simulink model "Top_Level"  (Simulink 7.5)
settings: Solver=ode45  StartTime=0.0  StopTime=inf  RelTol=1e-3
undefined symbols (not defined in the file): dfilt, DiscIntNeverNeededParam, fspecial, gray, Horn, imresize, Low, Rec, Schunck, SDTV
libraries: simulink x13, dspobslib x10, dspsigops x4, vipgeotforms x4, viptextngfix x4, vipsnks x3, dspmtrx3 x2, vipanalysis x2, vipconversions x1, dsparch4 x1, dspswit3 x1, vipsrcs x1
(part 2 of 2)

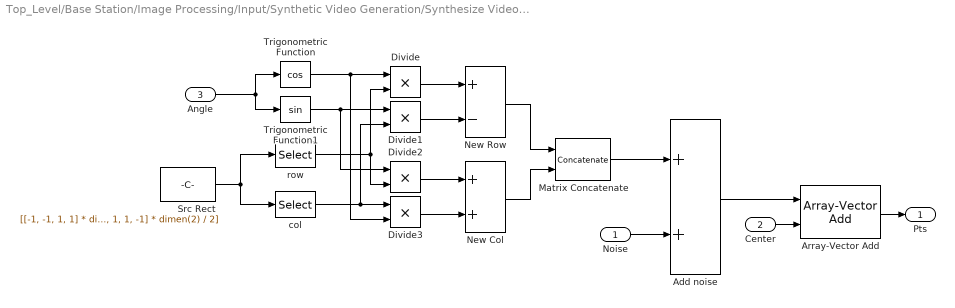
== system Top_Level/Base Station/Image Processing/Input/Synthetic Video Generation/Synthesize Video/Corner Locations ==
  Noise : Inport
  Center : Inport  Port=2
  Angle : Inport  Port=3
  Add noise : Sum  OutDataType=sfix(16)  OutScaling=2^-10
  Array-Vector Add : dspmtrx3/Array-Vector Add  DialogController=dspDDGCreate  DialogControllerArgs=DataTag2  Dimension=1  V_Source=Input port  V_VectFromMask=[0.5 0.25]  firstCoeffDataTypeStr=Inherit: Same word length as input  firstCoeffLastDataTypeStr=Inherit: Same word length as input  firstCoeffMin=[]  firstCoeffMax=[]  outputDataTypeStr=Inherit: Same as accumulator  outputLastDataTypeStr=Inherit: Same as accumulator  outputMin=[]  outputMax=[]  roundingMode=Floor  overflowMode=off
  Divide{,1..3} (4 alike) : Product  Inputs=**  OutDataType=sfix(16)  OutScaling=2^-10
  Matrix Concatenate : Concatenate  Mode=Multidimensional array
  New Col : Sum  OutDataType=sfix(16)  OutScaling=2^-10
  New Row : Sum  Inputs=+-  OutDataType=sfix(16)  OutScaling=2^-10
  Src Rect : Constant  Value=[[-1, -1, 1, 1] * dimen(1) / 2; [-1, 1, 1, -1] * dimen(2) / 2]  OutDataType=sfix(16)  OutScaling=2^0
  Trigonometric Function : Trigonometry  Operator=cos
  Trigonometric Function1 : Trigonometry
  col : Selector  NumberOfDimensions=2  IndexMode=Zero-based  InputPortWidth=3  IndexOptions=Index vector (dialog),Select all  Indices=1,1  OutputSizes=1,1
  row : Selector  NumberOfDimensions=2  IndexMode=Zero-based  InputPortWidth=3  IndexOptions=Index vector (dialog),Select all  Indices=0,1  OutputSizes=1,1
  Pts : Outport
  wires:
  Noise/1 -> Add noise/2
  Center/1 -> Array-Vector Add/2
  Array-Vector Add/1 -> Pts/1
  Src Rect/1 -> col/1, row/1
  Divide2/1 -> New Col/1
  Divide3/1 -> New Col/2
  New Row/1 -> Matrix Concatenate/1
  New Col/1 -> Matrix Concatenate/2
  Matrix Concatenate/1 -> Add noise/1
  Angle/1 -> Trigonometric Function/1, Trigonometric Function1/1
  Divide/1 -> New Row/1
  Divide1/1 -> New Row/2
  Trigonometric Function/1 -> Divide3/2, Divide/1
  Trigonometric Function1/1 -> Divide2/1, Divide1/1
  row/1 -> Divide2/2, Divide/2
  col/1 -> Divide1/2, Divide3/1
  Add noise/1 -> Array-Vector Add/1

== system Top_Level/Base Station/Image Processing/Mosaicking/Corner Matching/Calculate Distances/For Iterator Subsystem ==
  F1 : Inport  OutDataType=sfix(16)  OutScaling=2^0
  N1 : Inport  Port=2  OutDataType=sfix(16)  OutScaling=2^0
  F2 : Inport  Port=3  OutDataType=sfix(16)  OutScaling=2^0
  N2 : Inport  Port=4  OutDataType=sfix(16)  OutScaling=2^0
  For Iterator : ForIterator  IterationSource=external  IndexMode=Zero-based
  For Iterator Subsystem : Subsystem  TreatAsAtomicUnit=on
  Select feature  for 1 corner : Selector  NumberOfDimensions=2  IndexMode=Zero-based  InputPortWidth=2  IndexOptions=Select all,Index vector (port)  Indices=0,1  OutputSizes=1,1
  Update feature  for a corner : Assignment  NumberOfDimensions=2  IndexMode=Zero-based  OutputInitialize=Specify size for each dimension in table  IndexOptions=Assign all,Index vector (port)  Indices=1,1  OutputSizes=maxNum,maxNum
  Dis : Outport  OutDataType=sfix(16)  OutScaling=2^0
  wires:
  Update feature  for a corner/1 -> Dis/1
  N1/1 -> For Iterator Subsystem/2(N1)
  F1/1 -> For Iterator Subsystem/1(F1)
  Select feature  for 1 corner/1 -> For Iterator Subsystem/3(f2)
  F2/1 -> Select feature  for 1 corner/1
  For Iterator/1 -> Select feature  for 1 corner/2, Update feature  for a corner/2
  N2/1 -> For Iterator/1
  For Iterator Subsystem/1(Dis) -> Update feature  for a corner/1

== system Top_Level/Base Station/Image Processing/Mosaicking/Corner Matching/Calculate Features/Calculate Point Features ==
  note: Calculate feature for a corner.
  I : Inport
  Pts : Inport  Port=2
  Num : Inport  Port=3
  For Iterator : ForIterator  IterationSource=external  IndexMode=Zero-based
  Reshape : Reshape  OutputDimensionality=Column vector (2-D)
  Selector : Selector  NumberOfDimensions=2  IndexMode=Zero-based  InputPortWidth=3  IndexOptions=Starting index (port),Starting index (port)  Indices=[1 3],1  OutputSizes=winLen,winLen
  Selector1 : Selector  NumberOfDimensions=2  IndexMode=Zero-based  InputPortWidth=3  IndexOptions=Select all,Index vector (port)  Indices=[1 3],1  OutputSizes=9,9
  Selector2 : Selector  IndexMode=Zero-based  InputPortWidth=2  IndexOptions=Index vector (dialog)  Indices=0  OutputSizes=9
  Selector3 : Selector  IndexMode=Zero-based  InputPortWidth=2  IndexOptions=Index vector (dialog)  Indices=1  OutputSizes=9
  Update Feature  for a Corner : Assignment  NumberOfDimensions=2  IndexMode=Zero-based  OutputInitialize=Specify size for each dimension in table  IndexOptions=Assign all,Index vector (port)  Indices=1,1  OutputSizes=winLen^2,maxNum
  F : Outport
  wires:
  Selector3/1 -> Selector/3
  Selector2/1 -> Selector/2
  Num/1 -> For Iterator/1
  Update Feature  for a Corner/1 -> F/1
  Pts/1 -> Selector1/1
  I/1 -> Selector/1
  Reshape/1 -> Update Feature  for a Corner/1
  Selector/1 -> Reshape/1
  Selector1/1 -> Selector2/1, Selector3/1
  For Iterator/1 -> Update Feature  for a Corner/2, Selector1/2

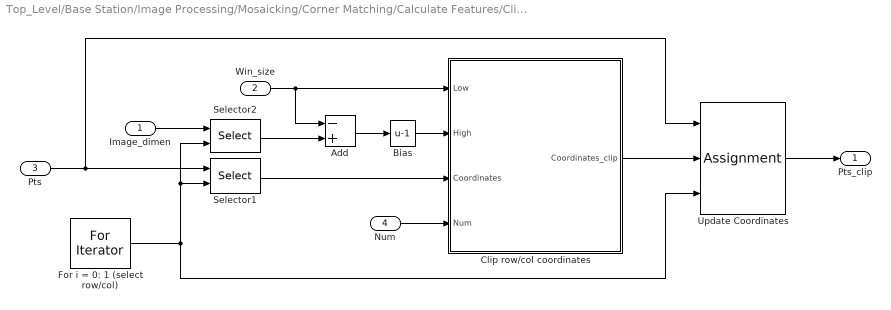
== system Top_Level/Base Station/Image Processing/Mosaicking/Corner Matching/Calculate Features/Clip Point Coordinates ==
  Image_dimen : Inport  OutDataType=sfix(16)  OutScaling=2^0
  Win_size : Inport  Port=2  OutDataType=sfix(16)  OutScaling=2^0
  Pts : Inport  Port=3
  Num : Inport  Port=4
  Add : Sum  Inputs=-+  OutDataType=sfix(16)  OutScaling=2^-10
  Bias : Bias  Bias=-1
  Clip row/col coordinates : Subsystem
  For i = 0: 1 (select row/col) : ForIterator  IterationLimit=2  IndexMode=Zero-based
  Selector1 : Selector  NumberOfDimensions=2  IndexMode=Zero-based  InputPortWidth=3  IndexOptions=Index vector (port),Select all  Indices=[1 3],1  OutputSizes=9,9
  Selector2 : Selector  IndexMode=Zero-based  InputPortWidth=2  IndexOptions=Index vector (port)  Indices=[1 3]  OutputSizes=9
  Update Coordinates : Assignment  NumberOfDimensions=2  IndexMode=Zero-based  IndexOptions=Index vector (port),Assign all  Indices=1,1  OutputSizes=81,50
  Pts_clip : Outport  OutDataType=sfix(16)  OutScaling=2^0
  wires:
  Selector2/1 -> Add/2
  For i = 0: 1 (select row/col)/1 -> Selector1/2, Selector2/2, Update Coordinates/3
  Clip row/col coordinates/1(Coordinates_clip) -> Update Coordinates/2
  Bias/1 -> Clip row/col coordinates/2(High)
  Update Coordinates/1 -> Pts_clip/1
  Num/1 -> Clip row/col coordinates/4(Num)
  Selector1/1 -> Clip row/col coordinates/3(Coordinates)
  Win_size/1 -> Add/1, Clip row/col coordinates/1(Low)
  Add/1 -> Bias/1
  Image_dimen/1 -> Selector2/1
  Pts/1 -> Update Coordinates/1, Selector1/1

== system Top_Level/Base Station/Image Processing/Input/Synthetic Video Generation/Synthesize Video/Center Locations/Saturate center coordinates ==
  Center : Inport
  Size : Inport  Port=2
  Center2 : Sum  Inputs=-+  OutDataType=sfix(16)  OutScaling=2^-10
  Min Dis to Boundary : Constant  Value=kron([ceil(sqrt(dimen(1)^2+dimen(2)^2)/2)], [1; 1])  OutDataType=sfix(16)  OutScaling=2^0
  MinMax : MinMax  Function=max  Inputs=2  OutDataType=sfix(16)  OutScaling=2^0
  MinMax1 : MinMax  Inputs=2  OutDataType=sfix(16)  OutScaling=2^0
  row1 : Selector  IndexMode=Zero-based  InputPortWidth=3  IndexOptions=Index vector (dialog)  Indices=[0 1]  OutputSizes=1
  Ctr : Outport
  wires:
  Size/1 -> row1/1
  MinMax1/1 -> Ctr/1
  Center/1 -> MinMax/1
  Center2/1 -> MinMax1/2
  MinMax/1 -> MinMax1/1
  row1/1 -> Center2/2
  Min Dis to Boundary/1 -> Center2/1, MinMax/2

== system Top_Level/Base Station/Image Processing/Mosaicking/Corner Matching/Calculate Distances/For Iterator Subsystem/For Iterator Subsystem ==
  F1 : Inport  OutDataType=sfix(16)  OutScaling=2^0
  N1 : Inport  Port=2  OutDataType=sfix(16)  OutScaling=2^0
  f2 : Inport  Port=3  OutDataType=sfix(16)  OutScaling=2^0
  Distance between two feature vectors : Subsystem
  For Iterator : ForIterator  IterationSource=external  IndexMode=Zero-based
  Select feature  for 1 corner : Selector  NumberOfDimensions=2  IndexMode=Zero-based  InputPortWidth=2  IndexOptions=Select all,Index vector (port)  Indices=0,1  OutputSizes=1,1
  Update feature  for a corner : Assignment  NumberOfDimensions=2  IndexMode=Zero-based  OutputInitialize=Specify size for each dimension in table  IndexOptions=Index vector (port),Assign all  Indices=1,1  OutputSizes=maxNum,1
  Dis : Outport  OutDataType=sfix(16)  OutScaling=2^0
  wires:
  Select feature  for 1 corner/1 -> Distance between two feature vectors/1(f1)
  f2/1 -> Distance between two feature vectors/2(f2)
  Update feature  for a corner/1 -> Dis/1
  F1/1 -> Select feature  for 1 corner/1
  For Iterator/1 -> Select feature  for 1 corner/2, Update feature  for a corner/2
  N1/1 -> For Iterator/1
  Distance between two feature vectors/1(dis) -> Update feature  for a corner/1

== system Top_Level/Base Station/Image Processing/Mosaicking/Corner Matching/Calculate Features/Clip Point Coordinates/Clip row/col coordinates ==
  Low : Inport  OutDataType=sfix(16)  OutScaling=2^0
  High : Inport  Port=2  OutDataType=sfix(16)  OutScaling=2^0
  Coordinates : Inport  Port=3
  Num : Inport  Port=4  OutDataType=sfix(16)  OutScaling=2^0
  Clip a Coordinate : Subsystem
  For Iterator : ForIterator  IterationSource=external  IterationLimit=2  IndexMode=Zero-based
  Select Coordinate of a Point : Selector  NumberOfDimensions=2  IndexMode=Zero-based  InputPortWidth=3  IndexOptions=Select all,Index vector (port)  Indices=[1 3],1  OutputSizes=9,1
  Update Feature  for a Corner : Assignment  NumberOfDimensions=2  IndexMode=Zero-based  IndexOptions=Assign all,Index vector (port)  Indices=1,1  OutputSizes=81,50
  Coordinates_clip : Outport  OutDataType=sfix(16)  OutScaling=2^0
  wires:
  Clip a Coordinate/1(Coordinate_clip) -> Update Feature  for a Corner/2
  Update Feature  for a Corner/1 -> Coordinates_clip/1
  High/1 -> Clip a Coordinate/2(High)
  Low/1 -> Clip a Coordinate/1(Low)
  Select Coordinate of a Point/1 -> Clip a Coordinate/3(Coordinate)
  Num/1 -> For Iterator/1
  Coordinates/1 -> Update Feature  for a Corner/1, Select Coordinate of a Point/1
  For Iterator/1 -> Select Coordinate of a Point/2, Update Feature  for a Corner/3

== system Top_Level/Base Station/Image Processing/Mosaicking/Corner Matching/Calculate Distances/For Iterator Subsystem/For Iterator Subsystem/Distance between two feature vectors ==
  f1 : Inport  OutDataType=sfix(16)  OutScaling=2^0
  f2 : Inport  Port=2  OutDataType=sfix(16)  OutScaling=2^0
  Abs : Abs  OutDataType=sfix(16)  OutScaling=2^0
  Add : Sum  Inputs=+-  OutDataType=sfix(16)  OutScaling=2^-10
  Sum of Elements : Sum  Inputs=+  OutDataType=sfix(16)  OutScaling=2^-10
  dis : Outport  OutDataType=sfix(16)  OutScaling=2^0
  wires:
  Sum of Elements/1 -> dis/1
  Abs/1 -> Sum of Elements/1
  Add/1 -> Abs/1
  f2/1 -> Add/2
  f1/1 -> Add/1

== system Top_Level/Base Station/Image Processing/Mosaicking/Corner Matching/Calculate Features/Clip Point Coordinates/Clip row/col coordinates/Clip a Coordinate ==
  Low : Inport  OutDataType=sfix(16)  OutScaling=2^0
  High : Inport  Port=2  OutDataType=sfix(16)  OutScaling=2^0
  Coordinate : Inport  Port=3  OutDataType=sfix(16)  OutScaling=2^0
  MinMax1 : MinMax  Function=max  Inputs=2  OutDataType=sfix(16)  OutScaling=2^0
  MinMax2 : MinMax  Inputs=2  OutDataType=sfix(16)  OutScaling=2^0
  Coordinate_clip : Outport  OutDataType=sfix(16)  OutScaling=2^0
  wires:
  MinMax2/1 -> Coordinate_clip/1
  High/1 -> MinMax2/2
  MinMax1/1 -> MinMax2/1
  Low/1 -> MinMax1/2
  Coordinate/1 -> MinMax1/1

== matlab function Base Station/Image Processing/Mosaicking/Optical Flow Lines1 ==
  data: InlPts1 input double; InlPts2 input double; dir_Vec output double
function dir_Vec  = CalcDistanceVect(InlPts1, InlPts2) 
% Generates the coordinate points of optical flow lines

% persistent first_time;
% persistent X;
% persistent Y;
% persistent RV;
% persistent CV;
% if isempty(first_time)
%     first_time     = 1;
%     %% user may change the following three parameters
%     borderOffset   = 1;
%     decimFactorRow = 1;
%     decimFactorCol = 1;    
%     %%
%     [R] = (size(InlPts1, 1)+size(InlPts2, 1))/2;
%     [C] = (size(InlPts1, 2)+size(InlPts2, 2))/2;
%     RV = borderOffset:decimFactorRow:(R-borderOffset);   
%     CV = borderOffset:decimFactorCol:(C-borderOffset);
%     [Y X] = meshgrid(CV,RV);
% end
% M = InlPts1;
% for i=1:size(InlPts1)
%   if (mod(i,2) == 0)
% 	M(1:1,:)=InlPts1(1:1,:);
%   else
%     M(1:1,:)=InlPts2(1:1,:);
%   end  
% end
dir_Vec = [InlPts1(1);InlPts2(1);InlPts1(2);InlPts2(2)];

== matlab function Base Station/Image Processing/Optical Flow/Optical Flow Lines1/Optical Flow Lines1 ==
  data: vel_Values input double; vel_Lines output double; dir_Vec output double; scaleFactor parameter double size=1
function [vel_Lines, dir_Vec]=OpticalFlowLines(vel_Values, scaleFactor) 

% Generates the coordinate points of optical flow lines

persistent first_time;
persistent X;
persistent Y;
persistent RV;
persistent CV;
if isempty(first_time)
    first_time     = 1;
    %% user may change the following three parameters
    borderOffset   = 5;
    decimFactorRow = 5;
    decimFactorCol = 5;    
    %%
    [R C] = size(vel_Values);
    RV = borderOffset:decimFactorRow:(R-borderOffset);   
    CV = borderOffset:decimFactorCol:(C-borderOffset);
    [Y X] = meshgrid(CV,RV);
end

tmp = vel_Values(RV,CV);
tmp = tmp.*(-1);
X(:)=180;Y(:)=180;
tmp=sum(tmp(:))/size(tmp(:), 2);
dir_Vec = scaleFactor*[real(tmp), imag(tmp)]
vel_Lines = [X(:)';Y(:)';X(:)'+imag(tmp(:))';Y(:)'+real(tmp(:))'];
